simulink model "suspension_automovil_simulink (1)"  (R2025a)
settings: Solver=VariableStepAuto  StartTime=0.0  StopTime=10.0  RelTol=1e-3
InitFcn:
  | m1=290;
  | b1=1000;
  | m2=59;
  | k1=16182;
  | f=0;
  | k2=19000;

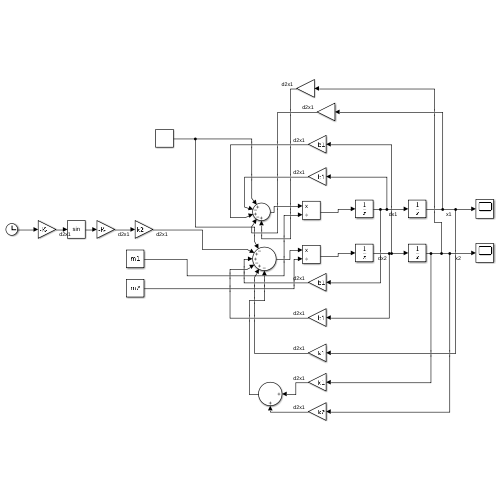
[thumbnail: Simulink's stored preview of the top-level diagram]
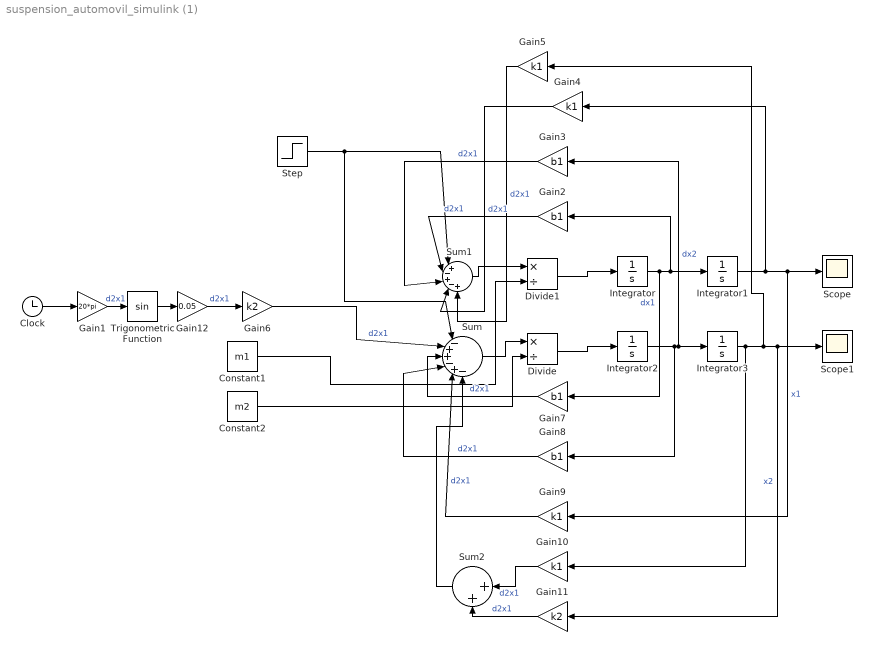
== system suspension_automovil_simulink (1) ==
  Clock : Clock
  Constant1 : Constant  Value=m1
  Constant2 : Constant  Value=m2
  Divide : Product  Inputs=*/
  Divide1 : Product  Inputs=*/
  Gain1 : Gain  Gain=20*pi
  Gain{4..5,9..10} (4 alike) : Gain  Gain=k1
  Gain11 : Gain  Gain=k2
  Gain12 : Gain  Gain=0.05
  Gain{2..3,7..8} (4 alike) : Gain  Gain=b1
  Gain6 : Gain  Gain=k2
  Integrator{,1..3} (4 alike) : Integrator
  Scope : Scope
      settings: ActiveDisplayYMinimum=-0.0045242196209999272  ActiveDisplayYMaximum=0.00559178283562917
  Scope1 : Scope
      settings: ActiveDisplayYMinimum=-0.008333043785775365  ActiveDisplayYMaximum=0.0135700887518613
  Step : Step  Before=f  After=0  SampleTime=0
  Sum : Sum  Inputs=|-++-+-
  Sum1 : Sum  Inputs=|+-+-+
  Sum2 : Sum  Inputs=|++
  Trigonometric Function : Trigonometry
  wires:
  Integrator1/1 -> Gain4/1, Gain9/1, Scope/1  "x1"
  Integrator3/1 -> Gain10/1, Gain5/1, Gain11/1, Scope1/1  "x2"
  Integrator2/1 -> Gain8/1, Gain3/1, Integrator3/1  "dx2"
  Integrator/1 -> Gain7/1, Gain2/1, Integrator1/1  "dx1"
  Step/1 -> Sum/1, Sum1/1
  Gain2/1 -> Sum1/2  "d2x1"
  Gain3/1 -> Sum1/3  "d2x1"
  Gain4/1 -> Sum1/4  "d2x1"
  Gain5/1 -> Sum1/5  "d2x1"
  Gain6/1 -> Sum/2  "d2x1"
  Gain7/1 -> Sum/3  "d2x1"
  Gain8/1 -> Sum/4  "d2x1"
  Gain9/1 -> Sum/5  "d2x1"
  Gain10/1 -> Sum2/1  "d2x1"
  Gain11/1 -> Sum2/2  "d2x1"
  Sum2/1 -> Sum/6
  Divide1/1 -> Integrator/1
  Sum1/1 -> Divide1/1
  Divide/1 -> Integrator2/1
  Sum/1 -> Divide/1
  Constant1/1 -> Divide1/2
  Constant2/1 -> Divide/2
  Gain1/1 -> Trigonometric Function/1  "d2x1"
  Trigonometric Function/1 -> Gain12/1
  Gain12/1 -> Gain6/1  "d2x1"
  Clock/1 -> Gain1/1
